simulink model "TestRocket_2026"  (R2025a)
settings: Solver=VariableStepAuto  StartTime=0.0  StopTime=54  RelTol=1e-3
libraries: aerolibasang x5, simulink_extras x2, aerolibanim x1, aerolibatmos2 x1
settings Model: Creator=Ranvir  LastModifiedBy=Ranvir
settings DebuggingCC: SignalInfNanChecking=error

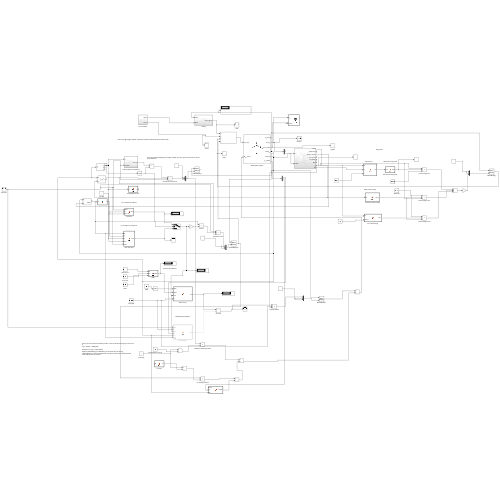
[thumbnail: Simulink's stored preview of the top-level diagram]
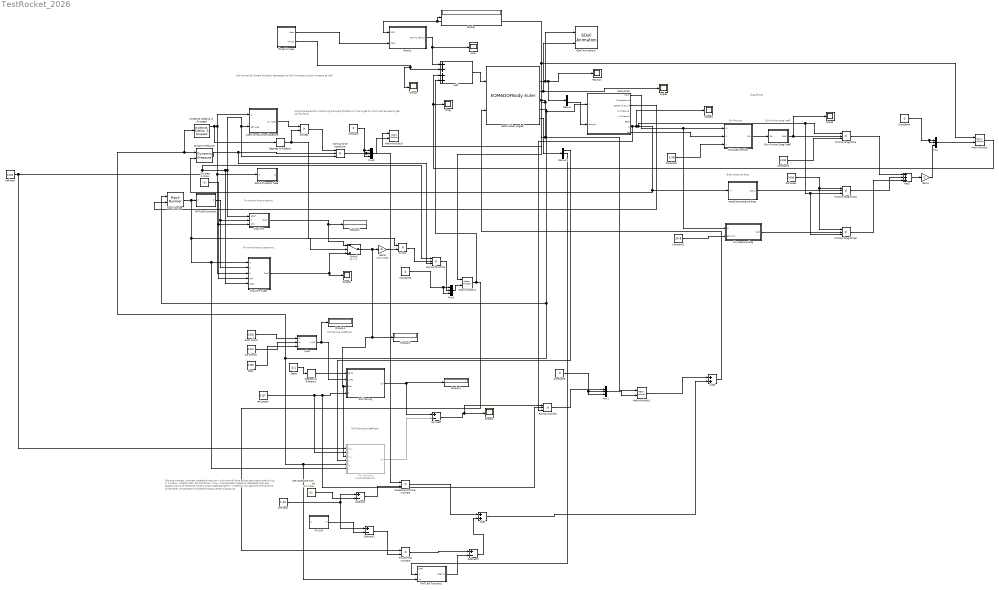
== system TestRocket_2026 ==
  note: drag forces
  note: 1
  note: Roll forcing Coefficent
  note: Fin normal force supersonic
  note: Using the equations multiplying the angle of attack by Cna to get Cn which can be used to get normal force
  note: Cna correct @ 0 angle of attack, decreases as AOA increases should increase as well
  note: Fin normal force subsonic
  note: Roll Damping Coefficent
  note: Skin friction
  note: Skin friction drag coeff
  note: Body pressure drag
  note: Pitching moment, moment created at position x with normal force acting upon nose cone tip
      | Xcg = Xcpress - stability*60?
      |
      | Normal force x (Xcg - XcpressNose)
      | Negative (destabalizing) pos Stabalizing vol of nosecone (prob wrong) 0.00221027027m^3 need to calculate the normal force of the other components first before finding center of pressure
  6DOF (Euler Angles) : EOM6DOFBodyEuler  mass_0=26.452  inertia=[6.531914 0 0; 0 6.531914 0; 0 0 0.635615]
  6DoF Animation1 : aerolibanim/6DoF Animation  u1=[0 4000 -2000 2000 -5000 -3000]  u2=0.1  u3=10  u4=[4000 0 -5000]  u5=Fixed position  u6=[2000 500 -3150]  u7=0.3  u8=on
  Add : Sum  Inputs=++++
  Add1 : Sum  Inputs=+++
  Add2 : Sum
  Add3 : Sum
  Angles : Scope
      settings: ActiveDisplayYMinimum=-4.5236731288085839  ActiveDisplayYMaximum=3.0954990419204327
  Cn fins : Product  Inputs=**
  Cna1 fins : MATLAB Function  TreatAsAtomicUnit=on
  Cna1 fins super : MATLAB Function  TreatAsAtomicUnit=on
  CoP body : Constant  Value=1.42
  CoP noseCone from tip : Constant  Value=0.177546
  Coeff normal force Nosecone : Subsystem
  Constant{,4..6} (4 alike) : Constant  Value=0
  Constant1 : Constant  Value=2.06
  Constant2 : Constant  Value=30.8
  Constant3 : Constant  Value=0.019
  Degrees to Radians : simulink_extras/Transformations/Degrees to Radians
  Degrees to Radians1 : simulink_extras/Transformations/Degrees to Radians
  Delta : Constant  Value=0.1
  Demux : Demux  Outputs=3
  Demux1 : Demux  Outputs=3
  Display{,1..4} (5 alike) : Display
  Divide1 : Product  Inputs=**
  Drag : Scope
      settings: ActiveDisplayYMinimum=-399.75467095348995  ActiveDisplayYMaximum=52.555641174970077  DataLoggingVariableName=ScopeData4
  Dynamic Pressure : aerolibasang/Dynamic Pressure
  Fin CoP : MATLAB Function  TreatAsAtomicUnit=on
  Fin area : Constant  Value=0.03344
  Fin pitching moment : Product  Inputs=**
  Fin pressure drag : MATLAB Function  TreatAsAtomicUnit=on
  Friction Drag force : Product  Inputs=***
  Friction Drag force1 : Product  Inputs=***
  Friction Drag force2 : Product  Inputs=***
  Gain1 : Gain  Gain=-1
  Gain3 : Gain  Gain=1.5*1.3406
  Grav : Scope
      settings: ActiveDisplayYMinimum=-10.132821204475356  ActiveDisplayYMaximum=5.5377021248938307  DataLoggingVariableName=ScopeData6
  Gravity : Subsystem
  "Incidence, Sideslip, & Airspeed" : aerolibasang/Incidence, Sideslip, & Airspeed
  MATLAB Function : MATLAB Function  TreatAsAtomicUnit=on
  MATLAB Function1 : MATLAB Function  TreatAsAtomicUnit=on
  MATLAB Function2 : MATLAB Function  TreatAsAtomicUnit=on
  Mach Number : aerolibasang/Mach Number
  MatrixMultiply{,1..3} (4 alike) : Product  Multiplication=Matrix(*)
  Mux{,1..3} (4 alike) : Mux  Inputs=3
  Normal force fins : Product  Inputs=***
  Normal force noseCone : Product  Inputs=***
  NoseCone pitching moment : Product  Inputs=**
  Position : Scope
      settings: ActiveDisplayYMinimum=-345.68920294660387  ActiveDisplayYMaximum=3111.2028265194353
  Ref area : Constant  Value=0.019
  Ref area1 : Constant  Value=0.019
  Roll Forcing : MATLAB Function  TreatAsAtomicUnit=on
  Roll damping : MATLAB Function  Commented=on  TreatAsAtomicUnit=on
  Rolling moment : Product  Inputs=***
  Root Chord : Constant  Value=0.318
  Scope{,1..3} (4 alike) : Scope
      Scope settings: ActiveDisplayYMinimum=0.076008560730816216  ActiveDisplayYMaximum=0.403028106514284  DataLoggingVariableName=ScopeData2
      Scope1 settings: ActiveDisplayYMinimum=63900.746660443481  ActiveDisplayYMaximum=67072.553717314237  DataLoggingVariableName=ScopeData3
      Scope2 settings: ActiveDisplayYMinimum=0.15600302895255286  ActiveDisplayYMaximum=0.15600506082886725  DataLoggingVariableName=ScopeData7
      Scope3 settings: ActiveDisplayYMinimum=-1.6378921729906146  ActiveDisplayYMaximum=15.489225016551334  DataLoggingVariableName=ScopeData8
  Skin Friction Drag Coeff : MATLAB Function  TreatAsAtomicUnit=on
  Span : Constant  Value=0.152
  Subsystem : Subsystem
  Subtract : Sum  Inputs=+-
  Subtract1 : Sum  Inputs=+-
  Subtract2 : Sum  Inputs=+-
  Switch : Switch  Criteria=u2 > Threshold  Threshold=1  SaturateOnIntegerOverflow=off  InputSameDT=off
  Thrust : Scope
      settings: ActiveDisplayYMinimum=-187.039604423378  ActiveDisplayYMaximum=1683.3564398104022  DataLoggingVariableName=ScopeData5
  Thrust & mass : Subsystem
  bodyLift Approx tube : MATLAB Function  TreatAsAtomicUnit=on
  noseCone pressure drag : MATLAB Function  TreatAsAtomicUnit=on
  ref Length : Constant  Value=0.157
  roll coeff : Sum  Inputs=+-
  tip Chord1 : Constant  Value=0.122
  yMac : MATLAB Function  TreatAsAtomicUnit=on
  wires:
  6DOF (Euler Angles)/4 -> MatrixMultiply3/1, MatrixMultiply2/1, MatrixMultiply1/1, MatrixMultiply/1, Display/1, Gravity/1(DCM)
  Thrust & mass/1(Mass) -> Gravity/2(Mass)
  Gravity/1(Gravity [Body]) -> Add/1, Grav/1
  Thrust & mass/2(Thrust) -> Thrust/1, Add/2
  Add/1 -> 6DOF (Euler Angles)/1
  6DOF (Euler Angles)/2 -> 6DoF Animation1/1, Demux/1, Position/1
  6DOF (Euler Angles)/3 -> 6DoF Animation1/2, Angles/1
  "Incidence, Sideslip, & Airspeed"/1 -> Cna1 fins super/3(a), bodyLift Approx tube/1(a), Coeff normal force Nosecone/1(a), Degrees to Radians/1
  Ref area/1 -> Roll damping/1(aRef), Normal force fins/1, Cna1 fins super/5(aRef), Normal force noseCone/3, Coeff normal force Nosecone/2(Ref Area), Cna1 fins/1(aRef)
  6DOF (Euler Angles)/5 -> Subsystem/1(V), Mach Number/1, "Incidence, Sideslip, & Airspeed"/1, Dynamic Pressure/1, MATLAB Function2/3(Vo), Roll damping/5(Vo)
  Subsystem/7(q) -> Rolling moment/3, Scope1/1, Friction Drag force2/3, Friction Drag force1/3, Friction Drag force/1, Dynamic Pressure/2, noseCone pressure drag/1(M)
  Dynamic Pressure/1 -> Normal force fins/3, Normal force noseCone/2
  Coeff normal force Nosecone/1(Cn nose) -> Divide1/1
  Divide1/1 -> Normal force noseCone/1
  Degrees to Radians/1 -> Cn fins/1, Divide1/2
  Subsystem/3(Speed of Sound) -> Mach Number/2
  Mach Number/1 -> Switch/2, Cna1 fins super/1(M), Roll damping/6(m), MATLAB Function1/1(m)
  MATLAB Function1/1(b) -> Cna1 fins super/2(b), Cna1 fins/2(b)
  Fin area/1 -> Cna1 fins super/4(aFin), Cna1 fins/3(aFin)
  Cna1 fins super/1(Cna1) -> Switch/3, Scope3/1
  Cna1 fins/1(Cna1) -> Switch/1, Display4/1
  Switch/1 -> Roll damping/3(Cna), Roll Forcing/3(Cna), Display3/1, Gain3/1
  Cn fins/1 -> Normal force fins/2
  ref Length/1 -> Roll damping/2(d), Rolling moment/2, Roll Forcing/4(d)
  Delta/1 -> Degrees to Radians1/1
  yMac/1(yMAC) -> Display2/1, Roll Forcing/2(yMac)
  Root Chord/1 -> yMac/1(Cr)
  tip Chord1/1 -> yMac/2(Ct)
  Span/1 -> yMac/3(s)
  6DOF (Euler Angles)/6 -> Demux1/1
  Demux1/1 -> Roll damping/4(W)
  Roll Forcing/1(Clf) -> roll coeff/1, Display1/1
  Roll damping/1(Cdf) -> roll coeff/2
  Demux/3 -> Subsystem/2(Height)
  Subsystem/8(Re) -> MATLAB Function/2(R)
  Constant1/1 -> MATLAB Function/3(L)
  Subsystem/1(Mach) -> Fin pressure drag/1(M), MATLAB Function/1(M)
  MATLAB Function/1(Cfc) -> Skin Friction Drag Coeff/1(Cfc)
  Constant2/1 -> Fin pressure drag/2(gamma)
  Skin Friction Drag Coeff/1(Cdsf) -> Scope/1, Friction Drag force/2
  Constant3/1 -> Friction Drag force/3
  Ref area1/1 -> Friction Drag force2/1, Friction Drag force1/1
  noseCone pressure drag/1(Cdp_n) -> Friction Drag force1/2
  Fin pressure drag/1(Cd_f) -> Friction Drag force2/2
  Friction Drag force/1 -> Add1/1
  Friction Drag force1/1 -> Add1/2
  Friction Drag force2/1 -> Add1/3
  Constant4/1 -> Mux/2, Mux/1
  Mux/1 -> MatrixMultiply/2
  MatrixMultiply/1 -> Add/3, Drag/1
  Add1/1 -> Gain1/1
  Gain1/1 -> Mux/3
  roll coeff/1 -> Rolling moment/1, Scope2/1
  Degrees to Radians1/1 -> Roll Forcing/1(delta)
  Gain3/1 -> Cn fins/2
  Constant5/1 -> Mux1/3, Mux1/2
  Mux1/1 -> MatrixMultiply1/2
  Rolling moment/1 -> Mux1/1
  Constant6/1 -> Mux2/3, Mux2/1
  Normal force fins/1 -> Mux2/2
  Mux2/1 -> MatrixMultiply2/2
  MatrixMultiply2/1 -> Add/4, Fin pitching moment/1
  CoP body/1 -> Subtract1/1, Subtract/1
  CoP noseCone from tip/1 -> Subtract/2
  Fin CoP/1(Xf) -> Subtract1/2
  Subtract/1 -> NoseCone pitching moment/2
  Subtract1/1 -> Fin pitching moment/2
  Normal force noseCone/1 -> NoseCone pitching moment/1, Mux3/2
  NoseCone pitching moment/1 -> Add2/1
  Add2/1 -> Add3/2
  Constant/1 -> Mux3/3, Mux3/1
  Mux3/1 -> MatrixMultiply3/2
  MatrixMultiply1/1 -> Add3/1
  Add3/1 -> 6DOF (Euler Angles)/2
  Fin pitching moment/1 -> Subtract2/1
  MATLAB Function2/1(Cdamp) -> Subtract2/2
  Subtract2/1 -> Add2/2
  Demux1/2 -> MATLAB Function2/2(w)

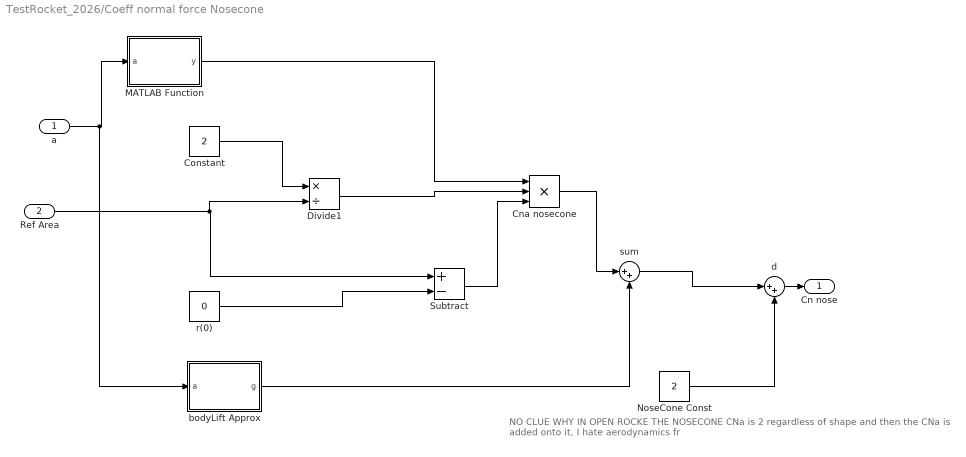
== system TestRocket_2026/Coeff normal force Nosecone ==
  note: NO CLUE WHY IN OPEN ROCKE THE NOSECONE CNa is 2 regardless of shape and then the CNa is added onto it, I hate aerodynamics fr
  a : Inport
  Ref Area : Inport  Port=2
  Cna nosecone : Product  Inputs=***
  Constant : Constant  Value=2
  Divide1 : Product  Inputs=*/
  MATLAB Function : MATLAB Function  TreatAsAtomicUnit=on
  NoseCone Const : Constant  Value=2
  Subtract : Sum  Inputs=+-
  bodyLift Approx : MATLAB Function  TreatAsAtomicUnit=on
  d : Sum  Inputs=|++
  r(0) : Constant  Value=0
  sum : Sum  Inputs=|++
  Cn nose : Outport
  wires:
  Ref Area/1 -> Divide1/2, Subtract/1
  Cna nosecone/1 -> sum/1
  sum/1 -> d/1
  Subtract/1 -> Cna nosecone/3
  bodyLift Approx/1(g) -> sum/2
  Constant/1 -> Divide1/1
  MATLAB Function/1(y) -> Cna nosecone/1
  a/1 -> bodyLift Approx/1(a), MATLAB Function/1(a)
  Divide1/1 -> Cna nosecone/2
  r(0)/1 -> Subtract/2
  NoseCone Const/1 -> d/2
  d/1 -> Cn nose/1

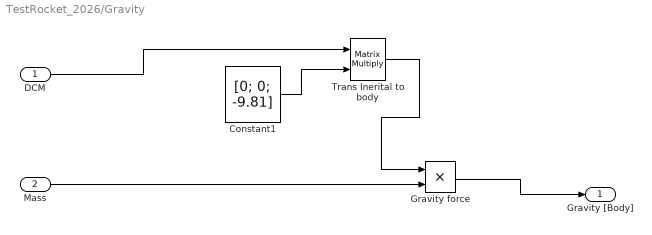
== system TestRocket_2026/Gravity ==
  DCM : Inport
  Mass : Inport  Port=2
  Constant1 : Constant  Value=[0; 0; -9.81]  VectorParams1D=off
  Gravity force : Product  Inputs=**
  Trans Inerital to body : Product  Multiplication=Matrix(*)
  Gravity [Body] : Outport
  wires:
  Constant1/1 -> Trans Inerital to body/2
  Trans Inerital to body/1 -> Gravity force/1
  Mass/1 -> Gravity force/2
  Gravity force/1 -> Gravity [Body]/1
  DCM/1 -> Trans Inerital to body/1

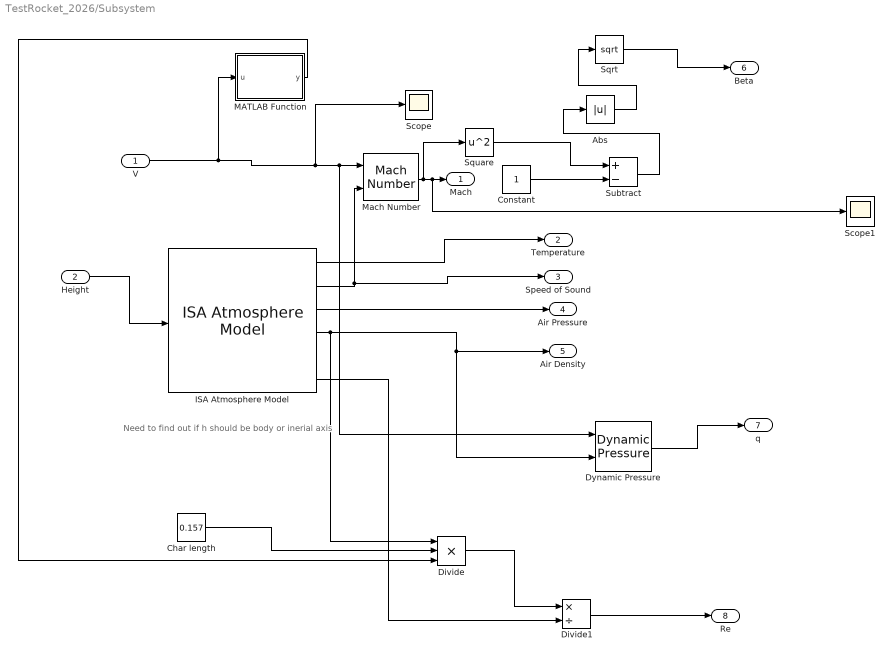
== system TestRocket_2026/Subsystem ==
  note: Need to find out if h should be body or inerial axis
  V : Inport
  Height : Inport  Port=2
  Abs : Abs  SaturateOnIntegerOverflow=off
  Char length : Constant  Value=0.157
  Constant : Constant
  Divide : Product  Inputs=***
  Divide1 : Product  Inputs=*/
  Dynamic Pressure : aerolibasang/Dynamic Pressure
  ISA Atmosphere Model : aerolibatmos2/ISA Atmosphere Model  useExtended=off  action=None  custom=off  viscosityOut=on  g=9.80665  gamma=1.4  R=287.0531  L=0.0065  h_trop=11000  h_strat=20000  rho0=1.225  P0=101325  T0=288.15  h0=0  S=110.4  Tref=273.15  muref=1.716e-5
  MATLAB Function : MATLAB Function  TreatAsAtomicUnit=on
  Mach Number : aerolibasang/Mach Number
  Scope : Scope
      settings: ActiveDisplayYMinimum=-1  ActiveDisplayYMaximum=1  DataLoggingVariableName=ScopeData9
  Scope1 : Scope
      settings: ActiveDisplayYMinimum=-0.075332759640287239  ActiveDisplayYMaximum=0.67799483676258532  DataLoggingVariableName=ScopeData10
  Sqrt : Sqrt
  Square : Math  Operator=square
  Subtract : Sum  Inputs=+-
  Mach : Outport
  Temperature : Outport  Port=2
  Speed of Sound : Outport  Port=3
  Air Pressure : Outport  Port=4
  Air Density : Outport  Port=5
  Beta : Outport  Port=6
  q : Outport  Port=7
  Re : Outport  Port=8
  wires:
  Mach Number/1 -> Square/1, Scope1/1, Mach/1
  Height/1 -> ISA Atmosphere Model/1
  ISA Atmosphere Model/2 -> Mach Number/2, Speed of Sound/1
  ISA Atmosphere Model/3 -> Air Pressure/1
  ISA Atmosphere Model/1 -> Temperature/1
  V/1 -> MATLAB Function/1(u), Scope/1, Dynamic Pressure/1, Mach Number/1
  ISA Atmosphere Model/4 -> Divide/1, Dynamic Pressure/2, Air Density/1
  Constant/1 -> Subtract/2
  Square/1 -> Subtract/1
  Subtract/1 -> Abs/1
  Abs/1 -> Sqrt/1
  Sqrt/1 -> Beta/1
  Dynamic Pressure/1 -> q/1
  Divide/1 -> Divide1/1
  ISA Atmosphere Model/6 -> Divide1/2
  Char length/1 -> Divide/2
  MATLAB Function/1(y) -> Divide/3
  Divide1/1 -> Re/1

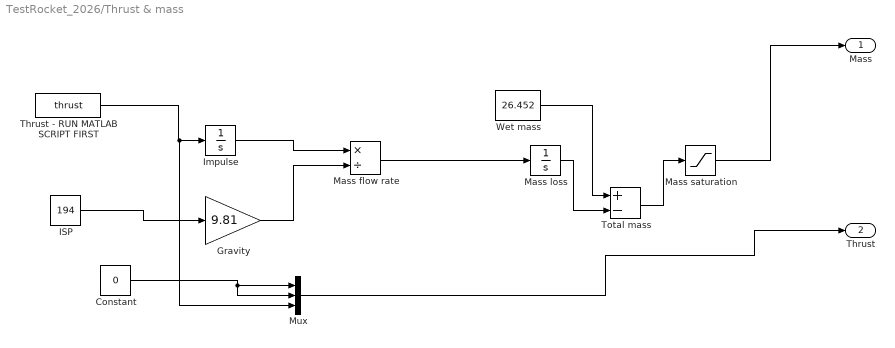
== system TestRocket_2026/Thrust & mass ==
  Constant : Constant  Value=0
  Gravity : Gain  Gain=9.81
  ISP : Constant  Value=194
  Impulse : Integrator
  Mass flow rate : Product  Inputs=*/
  Mass loss : Integrator  UpperSaturationLimit=7  LowerSaturationLimit=0
  Mass saturation : Saturate  UpperLimit=26.452  LowerLimit=19.536
  Mux : Mux  Inputs=3
  Thrust - RUN MATLAB SCRIPT FIRST : FromWorkspace  VariableName=thrust  OutputAfterFinalValue=Setting to zero
  Total mass : Sum  Inputs=+-
  Wet mass : Constant  Value=26.452
  Mass : Outport
  Thrust : Outport  Port=2
  wires:
  Thrust - RUN MATLAB SCRIPT FIRST/1 -> Mux/3, Impulse/1
  Total mass/1 -> Mass saturation/1
  Gravity/1 -> Mass flow rate/2
  Mass flow rate/1 -> Mass loss/1
  Wet mass/1 -> Total mass/1
  ISP/1 -> Gravity/1
  Impulse/1 -> Mass flow rate/1
  Mass loss/1 -> Total mass/2
  Mass saturation/1 -> Mass/1
  Constant/1 -> Mux/2, Mux/1
  Mux/1 -> Thrust/1

== matlab function TestRocket_2026/MATLAB Function ==
  data: M input; Cfc output; R input; L input
function Cfc = fcn(M,R, L)

Rs = 20;

Rcrit = 51*(Rs/L)^-1.039;


if R < 1*10^4
    Cfc = 1.48*10^-2;
elseif R < Rcrit
    cf = 1/((1.5*log(R) -5.6)^2);
    
    if M >= 1
        Cfc = cf/((1+0.15*M^2)^0.58);
    else
        Cfc = cf*(1-0.1*M^2);
    end

else
    cf = 0.032*(Rs/L)^0.2;

    if M >= 1
        Cfc = cf/(1+0.18*M^2);
    else
        Cfc = cf*(1-0.1*M^2);
    end

end

== matlab function TestRocket_2026/Skin Friction Drag Coeff ==
  data: Cfc input; Cdsf output
function Cdsf = fcn(Cfc)

fb =13.12101911;
Awb = 1.71841; % append to include nosecone surface area 
t =0.00686;
c= 0.0647;
AwF = 0.072381;
Aref = 0.157;

top1 = (1+1/(2*fb)*Awb);
top2 = (1+((2*t)/(c)))*AwF;

Cdsf = Cfc*((top1+top2))/Aref;

== matlab function TestRocket_2026/noseCone pressure drag ==
  data: M input; Cdp_n output
function Cdp_n = fcn(M)



Fn = 2.42;
epsilon = atan(1/(2*Fn));

if M > 1.3
    Cdp_n = 2.1*(sin(epsilon))^2 + 0.5*((sin(epsilon))/(sqrt(M^2-1)));
elseif M > 1
    Cdp_n =0.8*sin(deg2rad(30))^2;
elseif M == 1
    Cdp_n = sin(epsilon);
else 

    y1 =0.8*sin(deg2rad(30))^2;
    y2 = sin(epsilon);

    Cdp_n = (y1*(1.3 - M) + y2*(M-0))/(1.3);
    

end

== matlab function TestRocket_2026/Fin pressure drag ==
  data: M input; Cd_f output; gamma input
function Cd_f = fcn(M, gamma)


Cd_TE = 0; % assuming taper trailing edge

if M < 0.9
    Cd_LE = (1-M^2)^(-0.417) - 1;
elseif M>=0.9 && M<1
   Cd_LE = 1-1.785*(M-0.9);
else
    Cd_LE = 1.214-((0.502)/(M^2))+((0.1095)/(M^4));
end

Cd_LEgam = Cd_LE*(cosd(gamma))^2;

Cd_f = Cd_LEgam + Cd_TE;

== matlab function TestRocket_2026/Fin CoP ==
  data: M input; Xf output
function Xf = fcn(M)


S = 0.152;
aFin = 0.03344;

Ar = (2*S^2)/(aFin);

b = sqrt(abs(M^2-1));

arb = Ar*b;

C = 0.06472;


Xf = C*(((arb) - 0.67)/(2*arb - 1));

== matlab function TestRocket_2026/MATLAB Function2 ==
  data: aRef input; Cdamp output; w input; Vo input
function Cdamp = fcn(aRef, w,Vo)

v = norm(Vo);
d = 0.157;

zeta = 206-(31.8/2);

Cdamp = 0.6*((3*0.03344*zeta^3)/(aRef*d)) * (w^2/v^2);

== matlab function TestRocket_2026/Coeff normal force Nosecone/bodyLift Approx ==
  data: a input; g output
function g = fcn(a)

g = 1.1*(0.263603/0.019)*sind(a)^2;

== matlab function TestRocket_2026/Coeff normal force Nosecone/MATLAB Function ==
  data: a input; y output
function y = fcn(a)

if a == 0
    y = 1;
else
    y = sind(a)/a;
end

== matlab function TestRocket_2026/bodyLift Approx tube ==
  data: a input; g output
function g = fcn(a)

g = 1.1*(0.263603/0.019)*sind(a)^2;

== matlab function TestRocket_2026/Cna1 fins ==
  data: aRef input; Cna1 output; b input; aFin input
function Cna1 = fcn(aRef, b, aFin)

s = 0.152; %m^2
 %m^2
sA = 30.8; %deg


top = (2*pi) * ((s^2)/aRef);
fd = (b*s^2)/(aFin*cosd(sA)); 
bot = 1+sqrt(1+fd^2);


Cna1 = top/bot;

== matlab function TestRocket_2026/MATLAB Function1 ==
  data: m input; b output
function b = fcn(m)

b = sqrt(abs((m^2) - 1));

== matlab function TestRocket_2026/Cna1 fins super ==
  data: M input; b input; a input; aFin input; aRef input; Cna1 output
% function Cna1 = fcn(M, b, a, aFin, aRef)
% 
% gam = 1.4;
% gam1 = gam+1;
% 
% k1 = 2/b;
% k2 = (gam1*(M^4) -(4*b^2))/(4*b^4);
% k3 = ( (gam1*M^8)  + ((2*gam^2 - 7*gam - 5)*M^6) + 10*(gam1)*M^4 + 8)/(6*b^7);
% 
% 
% 
% 
% 
% 
% Cna1 = (aFin/aRef) *(k1 + k2*a + k3*a^2);


function Cna1 = fcn(M, b, a, aFin, aRef)

s = 0.152; %m^2
 %m^2
sA = 30.8; %deg


top = (2*pi) * ((s^2)/aRef);
fd = (b*s^2)/(aFin*cosd(sA)); 
bot = 1+sqrt(1+fd^2);


Cna1 = top/bot;

== matlab function TestRocket_2026/Roll Forcing ==
  data: delta input; yMac input; Clf output; Cna input; d input
function Clf = fcn(delta, yMac, Cna, d)

rt = 0.0785;
N = 3;

Clf = (N*(yMac + rt)*Cna*delta)/d;

== matlab function TestRocket_2026/yMac ==
  data: Cr input; yMAC output; Ct input; s input
function yMAC = fcn(Cr, Ct, s)




yMAC = (s/3) * ((Cr+2*Ct)/(Cr+Ct));

== matlab function TestRocket_2026/Roll damping ==
  data: aRef input; d input; Cna input; W input; Cdf output; Vo input; m input
function Cdf = fcn(aRef, d, Cna, W, Vo, m)

rt = 0.0785;
cr = 0.318;
ct = 0.122;
s = 0.152;

v = norm(Vo);

strip = (((cr+ct)/2)*rt^2*s) + (((cr+(2*ct))/3)*rt*s^2) + (((cr+(3*ct))/12)*s^3);

Cdf = 0.01;

if m >= 1
    Cdf = strip*((3)/(aRef*d));
elseif m < 1
    Cdf = strip*((3*Cna*W)/(aRef*d*v));
else
    Cdf =0.01;
end

== matlab function TestRocket_2026/Subsystem/MATLAB Function ==
  data: u input; y output
function y = fcn(u)

y = norm(u);
